simulink model "controlledsystem"  (R2016b)
settings: Solver=ode45  StartTime=0.0  StopTime=1  RelTol=1e-3  EnableMultiTasking=on
InitFcn:
  | clear all
  | ps=1e6;
  | pe=1;
  | Ap=5e-4;
  | V0=2e-3;
  | Vdead=10e-6;
  | Va0=Vdead;
  | Vb0=V0-Va0;
  | beta=1.71e9;
  | Cd=0.65;
  | w=25e-3;
  | ro=825.6;
  | m=1;
  | k=3e4;
  | b=6e2;
  | C1=1.5e-12;
  | Ki=14e-4;
  | Kd=1.2000e-007;
  | Kp=40e-2;
libraries: srolib x2
settings Model: Creator=COLONEL  LastModifiedBy=tapeltauer
settings DataIOCC: LimitDataPoints=on  SaveFormat=Array  SignalLoggingSaveFormat=ModelDataLogs
settings OptimizationCC: ExpressionDepthLimit=2147483647  InitFltsAndDblsToZero=on  LifeSpan=inf
settings DebuggingCC: UnderspecifiedInitializationDetection=Classic  MergeDetectMultiDrivingBlocksExec=none  SolverPrmCheckMsg=warning  FcnCallInpInsideContextMsg=warning  StateNameClashWarn=warning  StrictBusMsg=Warning  SFUnexpectedBacktrackingDiag=warning  SFNoUnconditionalDefaultTransitionDiag=warning  SFExecutionAtInitializationDiag=none
settings HardwareCC: ProdBitPerPointer=32  ProdBitPerSizeT=32  ProdBitPerPtrDiffT=32  ProdLargestAtomicFloat=None  ProdIntDivRoundTo=Undefined  ProdEndianess=Unspecified  ProdWordSize=32  ProdHWDeviceType=32-bit Generic
settings ModelReferenceCC: PropagateSignalLabelsOutOfModel=off
settings GRTTargetCC: TargetLangStandard=C89/C90 (ANSI)  CombineOutputUpdateFcns=off  GRTInterface=on
settings ConfigComp: CovMetricSettings=dw  CovHtmlReporting=on  CovSaveCumulativeToWorkspaceVar=on  CovSaveSingleToWorkspaceVar=on  CovExternalEMLEnable=off

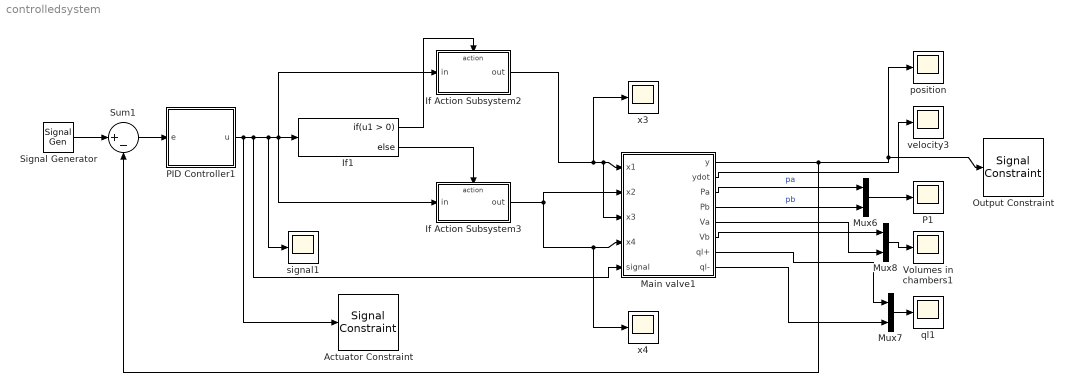
== system controlledsystem ==
  Actuator Constraint : srolib/Signal Constraint  SystemSampleTime=-1  DialogPosition=[0.0578125 0.1943359375 0.403125 0.2890625]  SaveIn=MAT file  SaveAs=controlledsystem_optim.mat  LogID=SRO_DataLog_1
  If Action Subsystem2 : Subsystem  TreatAsAtomicUnit=on
  If Action Subsystem3 : Subsystem  TreatAsAtomicUnit=on
  If1 : If
  Main valve1 : Subsystem
  Mux6 : Mux  Inputs=2
  Mux7 : Mux  Inputs=2
  Mux8 : Mux  Inputs=2
  Output Constraint : srolib/Signal Constraint  SystemSampleTime=-1  DialogPosition=[0.190625 0.119140625 0.3390625 0.259765625]  SaveIn=MAT file  SaveAs=controlledsystem_optim.mat  LogID=SRO_DataLog_2
  P1 : Scope
  PID Controller1 : Subsystem
  Signal Generator : SignalGenerator  WaveForm=square  Amplitude=1e-3  Frequency=5*pi  Units=rad/sec
  Sum1 : Sum  Inputs=|+-  SaturateOnIntegerOverflow=on
  Volumes in chambers1 : Scope
  position : Scope
  ql1 : Scope
  signal1 : Scope
  velocity3 : Scope
  x3 : Scope
  x4 : Scope
  wires:
  PID Controller1/1(u) -> If1/1, If Action Subsystem3/1(in), If Action Subsystem2/1(in), signal1/1, Main valve1/5(signal), Actuator Constraint/1
  If1/1 -> If Action Subsystem2/Action
  If1/2 -> If Action Subsystem3/Action
  If Action Subsystem3/1(out) -> Main valve1/2(x2), Main valve1/4(x4), x4/1
  Mux6/1 -> P1/1
  Main valve1/2(ydot) -> velocity3/1
  Mux8/1 -> Volumes in chambers1/1
  Main valve1/3(Pa) -> Mux6/1  "pa"
  Main valve1/4(Pb) -> Mux6/2  "pb"
  Main valve1/6(Vb) -> Mux8/1
  If Action Subsystem2/1(out) -> Main valve1/1(x1), Main valve1/3(x3), x3/1
  Main valve1/5(Va) -> Mux8/2
  Main valve1/7(ql+) -> Mux7/1
  Mux7/1 -> ql1/1
  Main valve1/8(ql-) -> Mux7/2
  Main valve1/1(y) -> Sum1/2, position/1, Output Constraint/1
  Sum1/1 -> PID Controller1/1(e)
  Signal Generator/1 -> Sum1/1

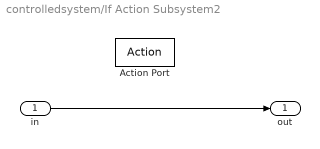
== system controlledsystem/If Action Subsystem2 ==
  in : Inport
  Action Port : ActionPort  ActionType=then
  out : Outport
  wires:
  in/1 -> out/1

== system controlledsystem/If Action Subsystem3 ==
  in : Inport
  Action Port : ActionPort  ActionType=else
  out : Outport
  wires:
  in/1 -> out/1

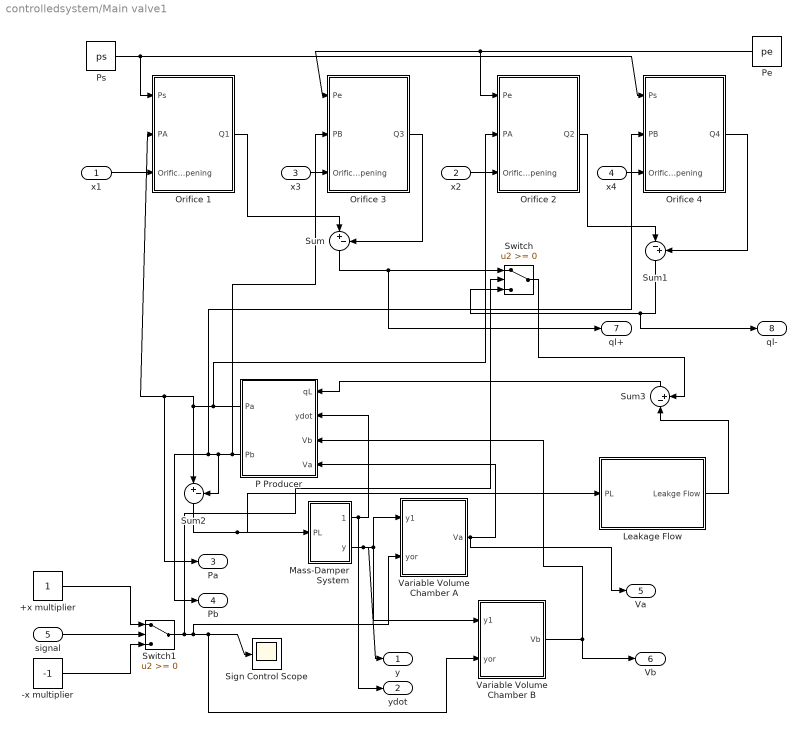
== system controlledsystem/Main valve1 ==
  x1 : Inport
  x2 : Inport  Port=2
  x3 : Inport  Port=3
  x4 : Inport  Port=4
  signal : Inport  Port=5
  +x multiplier : Constant
  -x multiplier : Constant  Value=-1
  Leakage Flow : Subsystem
  Mass-Damper System : Subsystem
  Orifice 1 : Subsystem
  Orifice 2 : Subsystem
  Orifice 3 : Subsystem
  Orifice 4 : Subsystem
  P Producer : Subsystem
  Pe : Constant  Value=pe
  Ps : Constant  Value=ps
  Sign Control Scope : Scope
  Sum : Sum  Inputs=|+-
  Sum1 : Sum  Inputs=|-+
  Sum2 : Sum  Inputs=|+-
  Sum3 : Sum  Inputs=|-+
  Switch : Switch
  Switch1 : Switch
  Variable Volume Chamber A : Subsystem
  Variable Volume Chamber B : Subsystem
  y : Outport
  ydot : Outport  Port=2
  Pa : Outport  Port=3
  Pb : Outport  Port=4
  Va : Outport  Port=5
  Vb : Outport  Port=6
  ql+ : Outport  Port=7
  ql- : Outport  Port=8
  wires:
  Orifice 1/1(Q1) -> Sum/1
  Orifice 2/1(Q2) -> Sum1/1
  Orifice 3/1(Q3) -> Sum/2
  Orifice 4/1(Q4) -> Sum1/2
  Sum/1 -> Switch/1, ql+/1
  P Producer/1(Pa) -> Orifice 1/2(PA), Pa/1, Sum2/1, Orifice 2/2(PA)
  P Producer/2(Pb) -> Orifice 3/2(PB), Sum2/2, Pb/1, Orifice 4/2(PB)
  Mass-Damper System/1(ydot) -> ydot/1, P Producer/2(ydot)
  Mass-Damper System/2(y) -> y/1, Variable Volume Chamber A/1(y1), Variable Volume Chamber B/1(y1)
  Ps/1 -> Orifice 1/1(Ps), Orifice 4/1(Ps)
  Pe/1 -> Orifice 2/1(Pe), Orifice 3/1(Pe)
  x1/1 -> Orifice 1/3(Orifice Opening)
  x2/1 -> Orifice 2/3(Orifice Opening)
  x3/1 -> Orifice 3/3(Orifice Opening)
  x4/1 -> Orifice 4/3(Orifice Opening)
  Sum1/1 -> Switch/3, ql-/1
  Switch/1 -> Sum3/2
  +x multiplier/1 -> Switch1/1
  Switch1/1 -> Switch/2, Variable Volume Chamber A/2(yor), Sign Control Scope/1, Variable Volume Chamber B/2(yor)
  -x multiplier/1 -> Switch1/3
  signal/1 -> Switch1/2
  Variable Volume Chamber A/1(Va) -> Va/1, P Producer/4(Va)
  Variable Volume Chamber B/1(Vb) -> P Producer/3(Vb), Vb/1
  Sum2/1 -> Mass-Damper System/1(PL), Leakage Flow/1(PL)
  Leakage Flow/1(Leakge Flow) -> Sum3/1
  Sum3/1 -> P Producer/1(qL)

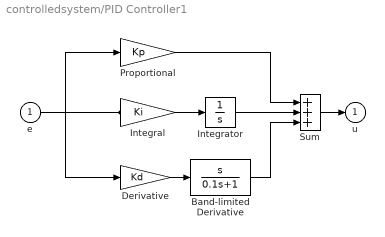
== system controlledsystem/PID Controller1 ==
  e : Inport
  Band-limited Derivative : TransferFcn  Numerator=[1 0]  Denominator=[0.1 1]
  Derivative : Gain  Gain=Kd  SaturateOnIntegerOverflow=on  OutDataTypeStr=Inherit: Same as input  ParamDataTypeStr=Inherit: Same as input
  Integral : Gain  Gain=Ki  SaturateOnIntegerOverflow=on  OutDataTypeStr=Inherit: Same as input  ParamDataTypeStr=Inherit: Same as input
  Integrator : Integrator
  Proportional : Gain  Gain=Kp  SaturateOnIntegerOverflow=on  OutDataTypeStr=Inherit: Same as input  ParamDataTypeStr=Inherit: Same as input
  Sum : Sum  Inputs=+++  SaturateOnIntegerOverflow=on  InputSameDT=on  OutDataTypeStr=Inherit: Same as first input
  u : Outport  InitialOutput=0
  wires:
  Integrator/1 -> Sum/2
  Derivative/1 -> Band-limited Derivative/1
  Sum/1 -> u/1
  e/1 -> Integral/1, Proportional/1, Derivative/1
  Band-limited Derivative/1 -> Sum/3
  Integral/1 -> Integrator/1
  Proportional/1 -> Sum/1

== system controlledsystem/Main valve1/Leakage Flow ==
  PL : Inport
  C1 : Gain  Gain=C1
  Leakge Flow : Outport
  wires:
  PL/1 -> C1/1
  C1/1 -> Leakge Flow/1

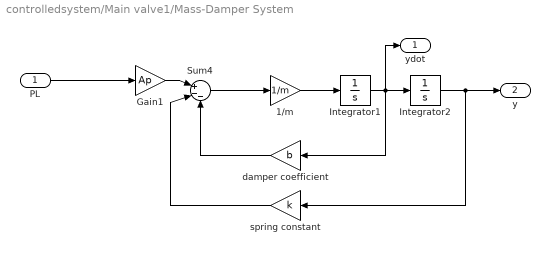
== system controlledsystem/Main valve1/Mass-Damper System ==
  PL : Inport
  1/m : Gain  Gain=1/m
  Gain1 : Gain  Gain=Ap
  Integrator1 : Integrator
  Integrator2 : Integrator
  Sum4 : Sum  Inputs=|+--
  damper coefficient : Gain  Gain=b
  spring constant : Gain  Gain=k
  ydot : Outport
  y : Outport  Port=2
  wires:
  Gain1/1 -> Sum4/1
  Sum4/1 -> 1/m/1
  1/m/1 -> Integrator1/1
  Integrator1/1 -> Integrator2/1, damper coefficient/1, ydot/1
  Integrator2/1 -> spring constant/1, y/1
  damper coefficient/1 -> Sum4/3
  spring constant/1 -> Sum4/2
  PL/1 -> Gain1/1

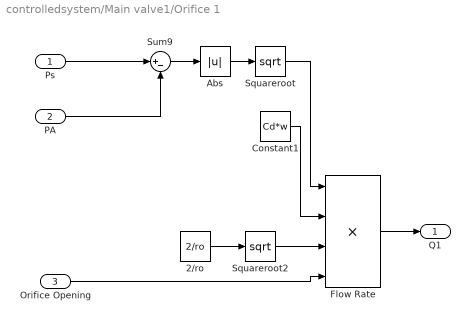
== system controlledsystem/Main valve1/Orifice 1 ==
  Ps : Inport
  PA : Inport  Port=2
  Orifice Opening : Inport  Port=3
  2/ro : Constant  Value=2/ro
  Abs : Abs
  Constant1 : Constant  Value=Cd*w
  Flow Rate : Product  Inputs=4  RndMeth=Zero
  Squareroot : Math  Operator=sqrt  SaturateOnIntegerOverflow=on
  Squareroot2 : Math  Operator=sqrt  SaturateOnIntegerOverflow=on
  Sum9 : Sum  Inputs=|+-
  Q1 : Outport
  wires:
  2/ro/1 -> Squareroot2/1
  Constant1/1 -> Flow Rate/2
  Sum9/1 -> Abs/1
  Abs/1 -> Squareroot/1
  Squareroot/1 -> Flow Rate/1
  Squareroot2/1 -> Flow Rate/3
  Orifice Opening/1 -> Flow Rate/4
  Flow Rate/1 -> Q1/1
  Ps/1 -> Sum9/1
  PA/1 -> Sum9/2

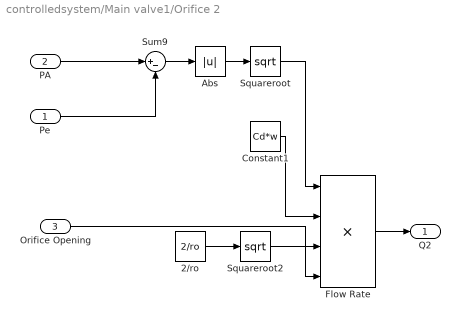
== system controlledsystem/Main valve1/Orifice 2 ==
  Pe : Inport
  PA : Inport  Port=2
  Orifice Opening : Inport  Port=3
  2/ro : Constant  Value=2/ro
  Abs : Abs
  Constant1 : Constant  Value=Cd*w
  Flow Rate : Product  Inputs=4  RndMeth=Zero
  Squareroot : Math  Operator=sqrt  SaturateOnIntegerOverflow=on
  Squareroot2 : Math  Operator=sqrt  SaturateOnIntegerOverflow=on
  Sum9 : Sum  Inputs=|+-
  Q2 : Outport
  wires:
  Flow Rate/1 -> Q2/1
  Squareroot2/1 -> Flow Rate/4
  Squareroot/1 -> Flow Rate/1
  Abs/1 -> Squareroot/1
  Sum9/1 -> Abs/1
  Constant1/1 -> Flow Rate/2
  2/ro/1 -> Squareroot2/1
  PA/1 -> Sum9/1
  Orifice Opening/1 -> Flow Rate/3
  Pe/1 -> Sum9/2

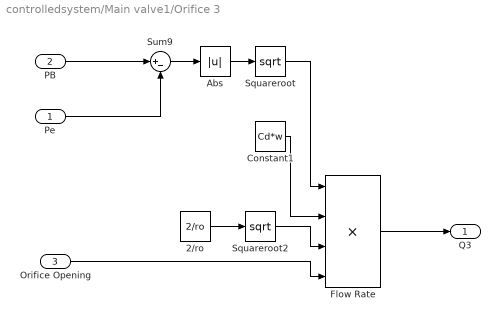
== system controlledsystem/Main valve1/Orifice 3 ==
  Pe : Inport
  PB : Inport  Port=2
  Orifice Opening : Inport  Port=3
  2/ro : Constant  Value=2/ro
  Abs : Abs
  Constant1 : Constant  Value=Cd*w
  Flow Rate : Product  Inputs=4  RndMeth=Zero
  Squareroot : Math  Operator=sqrt  SaturateOnIntegerOverflow=on
  Squareroot2 : Math  Operator=sqrt  SaturateOnIntegerOverflow=on
  Sum9 : Sum  Inputs=|+-
  Q3 : Outport
  wires:
  2/ro/1 -> Squareroot2/1
  Constant1/1 -> Flow Rate/2
  PB/1 -> Sum9/1
  Sum9/1 -> Abs/1
  Abs/1 -> Squareroot/1
  Squareroot/1 -> Flow Rate/1
  Squareroot2/1 -> Flow Rate/3
  Orifice Opening/1 -> Flow Rate/4
  Flow Rate/1 -> Q3/1
  Pe/1 -> Sum9/2

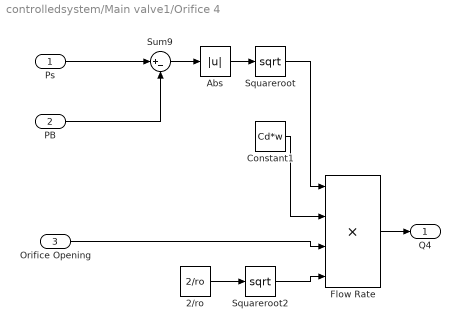
== system controlledsystem/Main valve1/Orifice 4 ==
  Ps : Inport
  PB : Inport  Port=2
  Orifice Opening : Inport  Port=3
  2/ro : Constant  Value=2/ro
  Abs : Abs
  Constant1 : Constant  Value=Cd*w
  Flow Rate : Product  Inputs=4  RndMeth=Zero
  Squareroot : Math  Operator=sqrt  SaturateOnIntegerOverflow=on
  Squareroot2 : Math  Operator=sqrt  SaturateOnIntegerOverflow=on
  Sum9 : Sum  Inputs=|+-
  Q4 : Outport
  wires:
  Flow Rate/1 -> Q4/1
  Squareroot2/1 -> Flow Rate/4
  Squareroot/1 -> Flow Rate/1
  Abs/1 -> Squareroot/1
  Sum9/1 -> Abs/1
  Constant1/1 -> Flow Rate/2
  2/ro/1 -> Squareroot2/1
  Orifice Opening/1 -> Flow Rate/3
  Ps/1 -> Sum9/1
  PB/1 -> Sum9/2

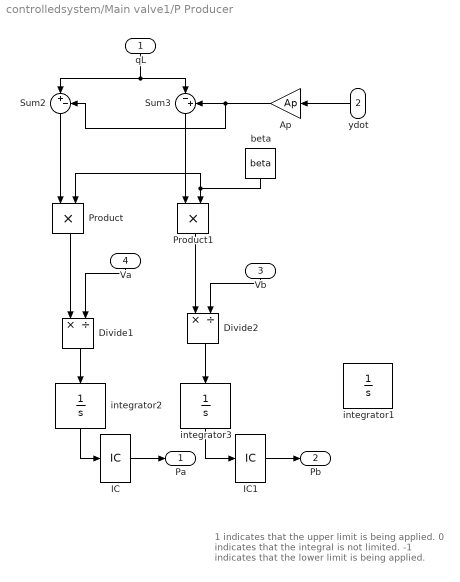
== system controlledsystem/Main valve1/P Producer ==
  note: 1 indicates that the upper limit is being applied.
      | 0 indicates that the integral is not limited.
      | -1 indicates that the lower limit is being applied.
  qL : Inport
  ydot : Inport  Port=2
  Vb : Inport  Port=3
  Va : Inport  Port=4
  Ap : Gain  Gain=Ap
  Divide1 : Product  Inputs=*/
  Divide2 : Product  Inputs=*/
  IC : InitialCondition  Value=ps/2
  IC1 : InitialCondition  Value=ps/2
  Product : Product  RndMeth=Zero
  Product1 : Product  RndMeth=Zero
  Sum2 : Sum  Inputs=|+-
  Sum3 : Sum  Inputs=|-+
  beta : Constant  Value=beta
  integrator1 : Integrator  ExternalReset=either  LimitOutput=on  UpperSaturationLimit=ps  LowerSaturationLimit=-1e-5  ShowSaturationPort=on  AbsoluteTolerance=ps
  integrator2 : Integrator  UpperSaturationLimit=ps  LowerSaturationLimit=-1e-5
  integrator3 : Integrator  UpperSaturationLimit=ps  LowerSaturationLimit=-1e-5
  Pa : Outport
  Pb : Outport  Port=2
  wires:
  qL/1 -> Sum3/1, Sum2/1
  Sum2/1 -> Product/1
  Divide1/1 -> integrator2/1
  Sum3/1 -> Product1/1
  Divide2/1 -> integrator3/1
  integrator2/1 -> IC/1
  Vb/1 -> Divide2/2
  Va/1 -> Divide1/2
  ydot/1 -> Ap/1
  Ap/1 -> Sum3/2, Sum2/2
  integrator3/1 -> IC1/1
  beta/1 -> Product1/2, Product/2
  Product/1 -> Divide1/1
  Product1/1 -> Divide2/1
  IC/1 -> Pa/1
  IC1/1 -> Pb/1

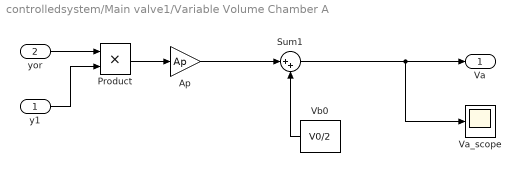
== system controlledsystem/Main valve1/Variable Volume Chamber A ==
  y1 : Inport
  yor : Inport  Port=2
  Ap : Gain  Gain=Ap
  Product : Product  RndMeth=Zero
  Sum1 : Sum  Inputs=|++
  Va_scope : Scope
  Vb0 : Constant  Value=V0/2
  Va : Outport
  wires:
  Sum1/1 -> Va/1, Va_scope/1
  Vb0/1 -> Sum1/2
  yor/1 -> Product/1
  y1/1 -> Product/2
  Ap/1 -> Sum1/1
  Product/1 -> Ap/1

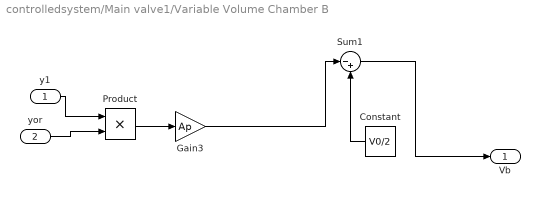
== system controlledsystem/Main valve1/Variable Volume Chamber B ==
  y1 : Inport
  yor : Inport  Port=2
  Constant : Constant  Value=V0/2
  Gain3 : Gain  Gain=Ap
  Product : Product  RndMeth=Zero
  Sum1 : Sum  Inputs=|-+
  Vb : Outport
  wires:
  Gain3/1 -> Sum1/1
  Constant/1 -> Sum1/2
  Sum1/1 -> Vb/1
  y1/1 -> Product/1
  yor/1 -> Product/2
  Product/1 -> Gain3/1
